simulink model "ee_motor_stepper_preparameterization"  (R2021a)
settings: Solver=ode23t  StartTime=0.0  StopTime=timeSimulation  FixedStep=0.001  MaxStep=1/(4*stepperMotorDriveData.microStep*f*4)  RelTol=1e-3  AbsTol=1e-3  EnableMultiTasking=on
PostLoadFcn:
  | ee_motor_stepper_preparameterization_data
StopFcn:
  | ee_addSimlogTimeStamp(bdroot)
undefined symbols (not defined in the file): CF, driveRampRate, f, loadTorque, stepperMotorData, stepperMotorDriveData, stepperMotorLoadData, tolerance
libraries: fl_lib x14, nesl_utility x5, simulink x1, ee_lib x1
CloseFcn:
  | try,close(figHandlePlotMotorPreparameterStepper),end
  | clear figHandlePlotMotorPreparameterStepper
  | 
  | try,close(figHandleMotorStepperPreparameter),end
  | clear figHandleMotorStepperPreparameter;
  | 
  | clear simlog_ee_motor_stepper_preparameterization;
  | 
  | clear voltageFactor userDefinedStepRate torqueTolerance
  | clear torque tolerance timeSimulation stepperMotorValue
  | clear  stepperMotorLoadData stepperMotorLoad stepperMotorDriveData
  | clear stepperMotorDrive stepperMotorData stepperMotor
  | clear slipped selectedStepRate numStep numRotation
  | clear notFinished nF modelStepper  modelInfo  modelFileName
  | clear loadTorqueLowInitial loadTorqueLow loadTorqueHighInitial loadTorqueHigh
  | clear loadTorque loadCycle i f driveRampRate  CF
  | clear blks name blockName blockNameParts
Description:
  | Pre-Parameterized Stepper Motor Block Validation
  | 
  | %
settings Model: Creator=The MathWorks, Inc.  LastModifiedBy=ssen
settings SolverCC: AlgebraicLoopSolver=TrustRegion
settings DataIOCC: MaxDataPoints=285000  SaveFormat=Array  SaveOutput=off  SignalLogging=off  DSMLogging=off  SaveTime=off  ReturnWorkspaceOutputs=off  SignalLoggingName=logsout_ee_motor_stepper_preparameterization
settings OptimizationCC: ExpressionDepthLimit=2147483647  InitFltsAndDblsToZero=on  LifeSpan=inf
settings DebuggingCC: UnderspecifiedInitializationDetection=Classic  MergeDetectMultiDrivingBlocksExec=none  FcnCallInpInsideContextMsg=warning  StateNameClashWarn=warning  PregeneratedLibrarySubsystemCodeDiagnostic=none  SFUnexpectedBacktrackingDiag=warning  SFNoUnconditionalDefaultTransitionDiag=warning  SFExecutionAtInitializationDiag=none  SFMachineParentedDataDiag=warning  ArithmeticOperatorsInVariantConditions=warning
settings HardwareCC: ProdBitPerPointer=32  ProdBitPerSizeT=32  ProdBitPerPtrDiffT=32  ProdLargestAtomicFloat=None  ProdIntDivRoundTo=Undefined  ProdEndianess=Unspecified  ProdWordSize=32  ProdHWDeviceType=32-bit Generic
settings ModelReferenceCC: PropagateSignalLabelsOutOfModel=off
settings SFSimCC: SimUseLocalCustomCode=off
settings RTWCC: RTWUseLocalCustomCode=off
settings CodeAppCC: StateflowObjectComments=on
settings GRTTargetCC: TargetLangStandard=C89/C90 (ANSI)  CombineOutputUpdateFcns=off  GRTInterface=on
settings ConfigComp: CovScope=ReferencedModels  CovMetricSettings=dw  CovSaveCumulativeToWorkspaceVar=on  CovSaveSingleToWorkspaceVar=on  CovExternalEMLEnable=off  CovSFcnEnable=off
settings SimscapeCC: SimscapeLogType=all  SimscapeLogSimulationStatistics=on  SimscapeLogName=simlog_ee_motor_stepper_preparameterization  SimscapeLogDataHistory=285000

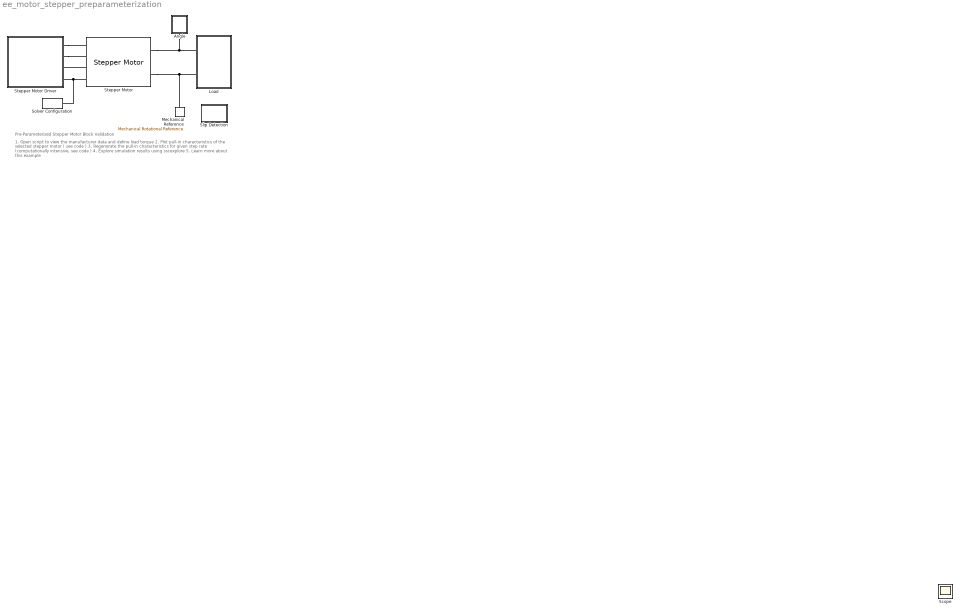
== system ee_motor_stepper_preparameterization ==
  note: 1. Open script to view the manufacturer data and define load torque
      | 2. Plot pull-in characteristics of the selected stepper motor ( see code )
      | 3. Regenerate the pull-in characteristics for given step rate (computationally intensive, see code )
      | 4. Explore simulation results using sscexplore
      | 5. Learn more about this example
  note: Pre-Parameterized Stepper Motor Block Validation
  Angle : Subsystem
  Load : Subsystem
  Mechanical Reference : fl_lib/Mechanical/Rotational Elements/Mechanical Rotational Reference
  Slip Detection : Subsystem
  Solver Configuration : nesl_utility/Solver Configuration  PhysicalDomain=network_engine_domain  SubClassName=solver  LeftPortType=input  RightPortType=generic  Tones=[]  Harmonics=[]  SimulateNoise=off  Profile=off  UseLocalSampling=off  EnableSwitchedLinearOptims=on  FrequencyDomain=off  UseCCode=off  RelTol=0.001  AbsTol=1e-06  MinStep=1e-09  ToWorkspace=off  RevertToSquareIcSolve=off  NumHomotopyIterations=100  PhasorMode=off  PhasorModeNumHarmonics=1  DoDC=off  ResidualTolerance=1e-9  UseLocalSolver=off  LocalSolverChoice=NE_BACKWARD_EULER_ADVANCER  LocalSolverSampleTime=.001  DoFixedCost=off  MaxNonlinIter=3  MaxModeIter=2  ComputeImpulses=off  ImpulseIterations=1  LinearAlgebra=auto  EquationFormulation=NE_TIME_EF  DelaysMemoryBudget=1024  AutomaticFiltering=off  FilteringTimeConstant=0.001  PartitionStorageMethod=AS_NEEDED  PartitionMemoryBudget=1024  PartitionMethod=FAST
      settings: SourceProductBaseCode=PW,SS
  Stepper Motor : ee_lib/Electromechanical/Reluctance & Stepper/Stepper Motor  Tag={'toolbox/physmod/elec/library/m/ee_lib_parts';'Electromechanical/Reluctance_and_Stepper/Stepper_Motor/Minebea/x08PM_K139BSTDCN.xml'}  step_or_av=1  w_vec=[0 1000 3000] rpm  T_vec=[2 2 1] N*m  assert_if_slipping=0  J_total=0.0001 kg*m^2  max_step_rate=10 Hz  Ra=6.5 Ohm  La=3.2 mH  Km=51.63 mN*m/A  Td=2.5 mN*m  Rm=Inf Ohm  Step=1.8 deg  J=2.9e-07 kg*m^2  B=2.65e-05 N*m/(rad/s)  speed0=0 rpm  theta0=0 deg  alpha=[0.00393 0.00393] 1/K  Tmeas=25 degC  T_vec2=[1.7 1.7 0.85] N*m  Tmeas2=125 degC  half_stepping=0  thermal_masses=[100 100] J/K  initial_temperatures=[25 25] degC  rotor_thermal_mass=50 J/K  rotor_initial_temperature=25 degC  Rm_percent_rotor=90
      settings: AttributesFormatString=Minebea:08PM-K139BSTDCN  SourceProductBaseCode=PS  InternalSimscapePortConfiguration="{\"Bottom\":[],\"Left\":[{\"id\":\"pA\",\"label\":\"A+\",\"type\":\"foundation.electrical.electrical\"},{\"id\":\"nA\",\"label\":\"A-\",\"type\":\"foundation.electrical.electrical\"},{\"id\":\"pB\",\"label\":\"B+\",\"type\":\"foundation.electrical.electrical\"},{\"id\":\"nB\",\"label\":\"B-\",\"type\":\"foundation.electrical.electrical\"}],\"Right\":[{\"id\":\"R\",\"label\":\"R\",\"type\":\"foundation.mechanical.rotational.rotational\"},{\"id\":\"C\",\"label\":\"C\",\"type\":\"foundation.mechanical.rotational.rotational\"}],\"Top\":[]}"
  Stepper Motor Driver : Subsystem
  Scope : Scope
  connections:
  Stepper Motor/RConn2 -- Mechanical Reference/LConn1 -- Load/LConn2
  Stepper Motor Driver/RConn1 -- Stepper Motor/LConn1
  Stepper Motor Driver/RConn2 -- Stepper Motor/LConn2
  Stepper Motor/LConn3 -- Stepper Motor Driver/RConn3
  Stepper Motor/LConn4 -- Solver Configuration/RConn1 -- Stepper Motor Driver/RConn4
  Stepper Motor/RConn1 -- Angle/LConn1 -- Load/LConn1

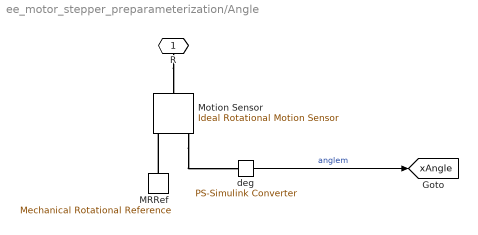
== system ee_motor_stepper_preparameterization/Angle ==
  MRRef : fl_lib/Mechanical/Rotational Elements/Mechanical Rotational Reference
  Motion Sensor : fl_lib/Mechanical/Mechanical Sensors/Ideal Rotational Motion Sensor  wrap_angle=simscape.enum.onoff.off  offset=0 rad
  deg : nesl_utility/PS-Simulink Converter  PhysicalDomain=network_engine_domain  SubClassName=ps_output  LeftPortType=input  RightPortType=output  PseudoPeriodic=off  Frequencies=[]  Unit=deg  AffineConversion=off
      settings: SourceProductBaseCode=PW,SS
  R : PMIOPort  Side=Left
  tag scope: xAngle=global
  wires:
  deg/1 -> [xAngle]  "anglem"
  connections:
  R/RConn1 -- Motion Sensor/LConn1
  Motion Sensor/RConn3 -- deg/LConn1
  MRRef/LConn1 -- Motion Sensor/RConn1

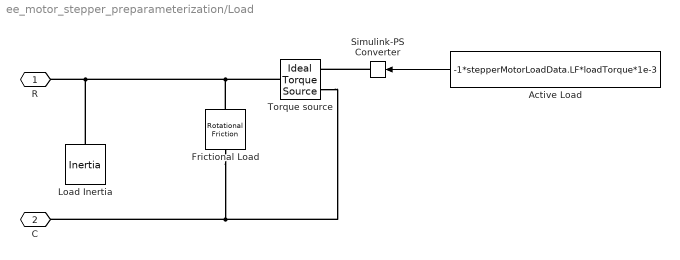
== system ee_motor_stepper_preparameterization/Load ==
  Active Load : Constant  Value=-1*stepperMotorLoadData.LF*loadTorque*1e-3
  Frictional Load : fl_lib/Mechanical/Rotational Elements/Rotational Friction  brkwy_trq=stepperMotorLoadData.loadDamping+1.005*loadTorque*(1-stepperMotorLoadData.LF)*1e-3+1e-8 N*m  brkwy_vel=0.01 rad/s  Col_trq=stepperMotorLoadData.loadDamping+loadTorque*(1-stepperMotorLoadData.LF)*1e-3+0.7e-8 N*m  visc_coef=(1e-9)*(1-stepperMotorLoadData.LF)+0*0.001*(loadTorque+stepperMotorLoadData.loadDamping)*(1-stepperMotorLoadData.LF)*1e-3/(f*4*stepperMotorData.Step*pi/180) N*m/(rad/s)  w_specify=on  w_priority=None  w=stepperMotorData.speed0 rpm  w_nominal_specify=off  w_nominal_unit=rad/s  w_nominal_value=1  t_specify=off  t_priority=None  t=0 N*m  t_nominal_specify=off  t_nominal_unit=N*m  t_nominal_value=1
  Load Inertia : fl_lib/Mechanical/Rotational Elements/Inertia  inertia=stepperMotorLoadData.loadInertia kg*m^2  num_ports=foundation.enum.numPorts2.one  w_specify=on  w_priority=High  w=stepperMotorData.speed0 rpm  w_nominal_specify=off  w_nominal_unit=rad/s  w_nominal_value=1  t_specify=off  t_priority=None  t=0 N*m  t_nominal_specify=off  t_nominal_unit=N*m  t_nominal_value=1
  Simulink-PS Converter : nesl_utility/Simulink-PS Converter  PhysicalDomain=network_engine_domain  SubClassName=ps_input  LeftPortType=input  RightPortType=output  PseudoPeriodic=off  Frequencies=[]  NoiseDistribution=none  NoiseParameters=[]  Unit=1  AffineConversion=off  FilteringAndDerivatives=provide  SimscapeFilterOrder=1  InputFilterTimeConstant=0.001  UdotUserProvided=0
      settings: SourceProductBaseCode=PW,SS
  Torque source : fl_lib/Mechanical/Mechanical Sources/Ideal Torque Source
  R : PMIOPort  Side=Left
  C : PMIOPort  Port=2  Side=Left
  wires:
  Active Load/1 -> Simulink-PS Converter/1
  connections:
  Torque source/RConn2 -- C/RConn1 -- Frictional Load/RConn1
  Torque source/LConn1 -- Load Inertia/LConn1 -- R/RConn1 -- Frictional Load/LConn1
  Simulink-PS Converter/RConn1 -- Torque source/RConn1

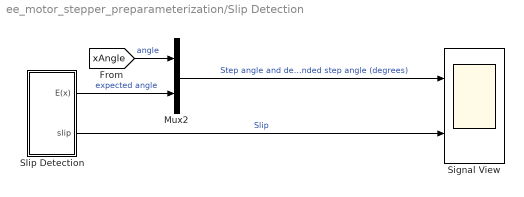
== system ee_motor_stepper_preparameterization/Slip Detection ==
  Mux2 : Mux  Inputs=2
  Signal View : Scope  NumInputPorts=2
  Slip Detection : Subsystem
  wires:
  [xAngle] -> Mux2/1  "angle"
  Mux2/1 -> Signal View/1  "Step angle and demanded step angle (degrees)"
  Slip Detection/1(E(x)) -> Mux2/2  "expected angle"
  Slip Detection/2(slip) -> Signal View/2  "Slip"

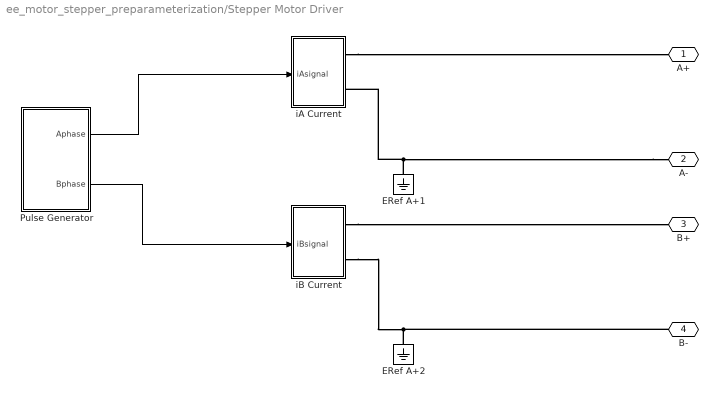
== system ee_motor_stepper_preparameterization/Stepper Motor Driver ==
  ERef A+1 : fl_lib/Electrical/Electrical Elements/Electrical Reference
  ERef A+2 : fl_lib/Electrical/Electrical Elements/Electrical Reference
  Pulse Generator : Subsystem
  iA Current : Subsystem
  iB Current : Subsystem
  A+ : PMIOPort  Side=Right
  A- : PMIOPort  Port=2  Side=Right
  B+ : PMIOPort  Port=3  Side=Right
  B- : PMIOPort  Port=4  Side=Right
  wires:
  Pulse Generator/2(Bphase) -> iB Current/1(iBsignal)
  Pulse Generator/1(Aphase) -> iA Current/1(iAsignal)
  connections:
  B-/RConn1 -- ERef A+2/LConn1 -- iB Current/RConn2
  iB Current/RConn1 -- B+/RConn1
  iA Current/RConn1 -- A+/RConn1
  A-/RConn1 -- ERef A+1/LConn1 -- iA Current/RConn2

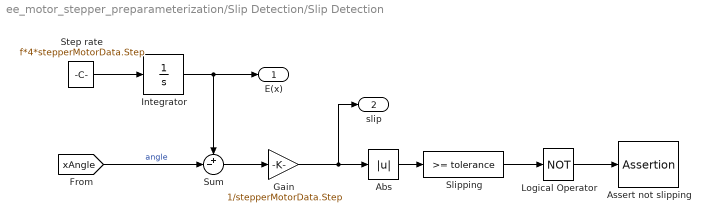
== system ee_motor_stepper_preparameterization/Slip Detection/Slip Detection ==
  Abs : Abs  ZeroCross=off
  Assert not slipping : Assertion  AssertionFailFcn=disp('Stepper slipped')
  Gain : Gain  Gain=1/stepperMotorData.Step
  Integrator : Integrator
  Logical Operator : Logic  Operator=NOT  AllPortsSameDT=off  OutDataTypeStr=boolean
  Slipping : simulink/Logic and Bit Operations/Compare To Constant  relop=>=  const=tolerance  OutDataTypeStr=boolean
  Step rate : Constant  Value=f*4*stepperMotorData.Step
  Sum : Sum  Inputs=+-|
  E(x) : Outport  VectorParamsAs1DForOutWhenUnconnected=off
  slip : Outport  Port=2  VectorParamsAs1DForOutWhenUnconnected=off
  wires:
  Step rate/1 -> Integrator/1
  Integrator/1 -> Sum/1, E(x)/1
  [xAngle] -> Sum/2  "angle"
  Gain/1 -> slip/1, Abs/1
  Slipping/1 -> Logical Operator/1
  Logical Operator/1 -> Assert not slipping/1
  Sum/1 -> Gain/1
  Abs/1 -> Slipping/1

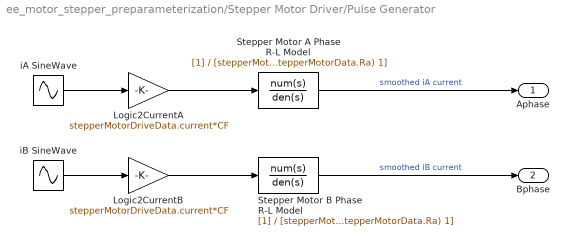
== system ee_motor_stepper_preparameterization/Stepper Motor Driver/Pulse Generator ==
  Logic2CurrentA : Gain  Gain=stepperMotorDriveData.current*CF
  Logic2CurrentB : Gain  Gain=stepperMotorDriveData.current*CF
  Stepper Motor A Phase R-L Model : TransferFcn  Denominator=[stepperMotorData.La*1e-3/(driveRampRate*stepperMotorData.Ra) 1]
  Stepper Motor B Phase R-L Model : TransferFcn  Denominator=[stepperMotorData.La*1e-3/(driveRampRate*stepperMotorData.Ra) 1]
  iA SineWave : Sin  Frequency=2*pi*f  Phase=pi/2  SampleTime=1/(f*4*stepperMotorDriveData.microStep)
  iB SineWave : Sin  Frequency=2*pi*f  SampleTime=1/(f*4*stepperMotorDriveData.microStep)
  Aphase : Outport  VectorParamsAs1DForOutWhenUnconnected=off
  Bphase : Outport  Port=2  VectorParamsAs1DForOutWhenUnconnected=off
  wires:
  iA SineWave/1 -> Logic2CurrentA/1
  iB SineWave/1 -> Logic2CurrentB/1
  Stepper Motor A Phase R-L Model/1 -> Aphase/1  "smoothed iA current"
  Stepper Motor B Phase R-L Model/1 -> Bphase/1  "smoothed iB current"
  Logic2CurrentA/1 -> Stepper Motor A Phase R-L Model/1
  Logic2CurrentB/1 -> Stepper Motor B Phase R-L Model/1

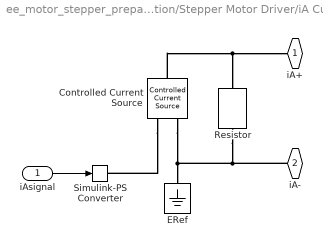
== system ee_motor_stepper_preparameterization/Stepper Motor Driver/iA Current ==
  iAsignal : Inport
  Controlled Current Source : fl_lib/Electrical/Electrical Sources/Controlled Current Source
  ERef : fl_lib/Electrical/Electrical Elements/Electrical Reference
  Resistor : fl_lib/Electrical/Electrical Elements/Resistor  R=stepperMotorData.Ra*2000 Ohm  i_specify=off  i_priority=None  i=0 A  i_nominal_specify=off  i_nominal_unit=A  i_nominal_value=1  v_specify=off  v_priority=None  v=0 V  v_nominal_specify=off  v_nominal_unit=V  v_nominal_value=1
  Simulink-PS Converter : nesl_utility/Simulink-PS Converter  PhysicalDomain=network_engine_domain  SubClassName=ps_input  LeftPortType=input  RightPortType=output  PseudoPeriodic=off  Frequencies=[]  NoiseDistribution=none  NoiseParameters=[]  Unit=A  AffineConversion=off  FilteringAndDerivatives=zero  SimscapeFilterOrder=1  InputFilterTimeConstant=.001  UdotUserProvided=0
      settings: SourceProductBaseCode=PW,SS
  iA+ : PMIOPort  Side=Right
  iA- : PMIOPort  Port=2  Side=Right
  wires:
  iAsignal/1 -> Simulink-PS Converter/1
  connections:
  Controlled Current Source/LConn1 -- iA+/RConn1 -- Resistor/LConn1
  iA-/RConn1 -- Resistor/RConn1 -- Controlled Current Source/RConn2 -- ERef/LConn1
  Controlled Current Source/RConn1 -- Simulink-PS Converter/RConn1

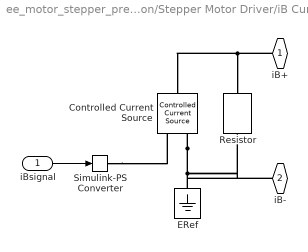
== system ee_motor_stepper_preparameterization/Stepper Motor Driver/iB Current ==
  iBsignal : Inport
  Controlled Current Source : fl_lib/Electrical/Electrical Sources/Controlled Current Source
  ERef : fl_lib/Electrical/Electrical Elements/Electrical Reference
  Resistor : fl_lib/Electrical/Electrical Elements/Resistor  R=stepperMotorData.Ra*2000 Ohm  i_specify=off  i_priority=None  i=0 A  i_nominal_specify=off  i_nominal_unit=A  i_nominal_value=1  v_specify=off  v_priority=None  v=0 V  v_nominal_specify=off  v_nominal_unit=V  v_nominal_value=1
  Simulink-PS Converter : nesl_utility/Simulink-PS Converter  PhysicalDomain=network_engine_domain  SubClassName=ps_input  LeftPortType=input  RightPortType=output  PseudoPeriodic=off  Frequencies=[]  NoiseDistribution=none  NoiseParameters=[]  Unit=A  AffineConversion=off  FilteringAndDerivatives=zero  SimscapeFilterOrder=1  InputFilterTimeConstant=.001  UdotUserProvided=0
      settings: SourceProductBaseCode=PW,SS
  iB+ : PMIOPort  Side=Right
  iB- : PMIOPort  Port=2  Side=Right
  wires:
  iBsignal/1 -> Simulink-PS Converter/1
  connections:
  Controlled Current Source/RConn2 -- iB-/RConn1 -- Resistor/RConn1 -- ERef/LConn1
  iB+/RConn1 -- Resistor/LConn1 -- Controlled Current Source/LConn1
  Simulink-PS Converter/RConn1 -- Controlled Current Source/RConn1
